simulink model "sampleModel1679"  (R2023a)
settings: Solver=VariableStepAuto  StartTime=0.0  StopTime=10.0  RelTol=1e-3
libraries: hdlsllib x5, simulink x2
settings Model: Creator=user1  LastModifiedBy=user1

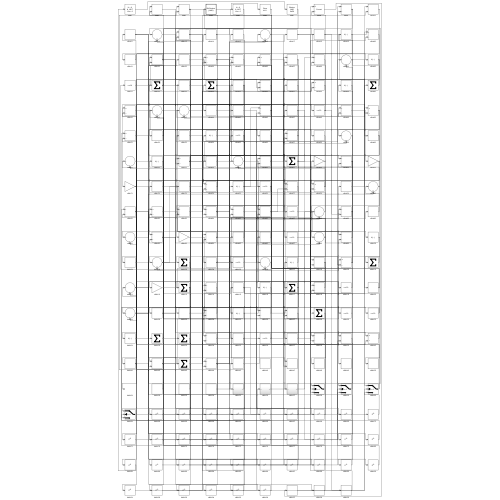
[thumbnail: Simulink's stored preview of the top-level diagram]
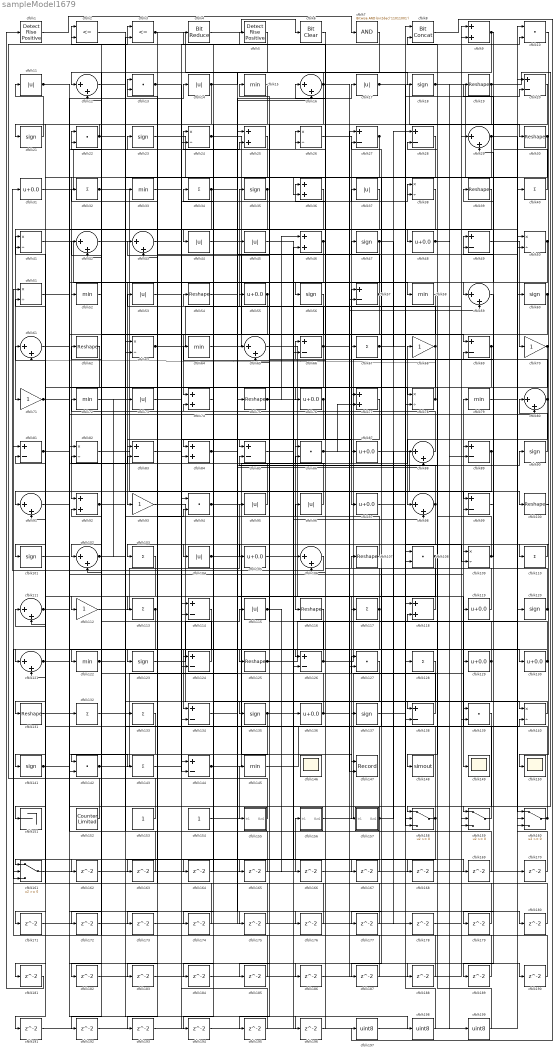
== system sampleModel1679 ==
  cfblk1 : hdlsllib/Logic and Bit Operations/Detect Rise Positive  vinit=0  OutDataTypeStr=boolean
  cfblk{10,13,22,86,94,108,127,139,142} (9 alike) : DotProduct  OutDataTypeStr=Inherit: Inherit via internal rule
  cfblk{19,30,39,54,62,75,100,107,116,125,131} (11 alike) : Reshape
  cfblk{18,21,23,35,47,56,60,90,101,120,123,135,137,141} (14 alike) : Signum
  cfblk{12,16,29,42..43,59,61,65,80,88,91,98,102,106,111,121} (16 alike) : Sum  Inputs=|++
  cfblk{32,34,40,67,103,110,113,117,128,132..133,143} (12 alike) : Sum  Inputs=+
  cfblk{11,14,17,37,44..45,53,73,95..96,104,115} (12 alike) : Abs  SaturateOnIntegerOverflow=off
  cfblk{31,48,55,76,87,97,105,119,129..130,136} (11 alike) : Bias  Bias=0.0  SaturateOnIntegerOverflow=off
  cfblk{24,26,38,41,50..51,63,78,82,109,140} (11 alike) : Product  Inputs=*/  RndMeth=Zero  SaturateOnIntegerOverflow=on
  cfblk{68,70..71,93,112} (5 alike) : Gain
  cfblk{20,27..28,49,57,66,69,81,83,85,89,99,114,124,126,134,138,144} (18 alike) : Sum  Inputs=+-
  cfblk{9,25,36,46,74,77,84,92,118} (9 alike) : Sum
  cfblk{15,33,52,58,64,72,79,122,145} (9 alike) : MinMax
  cfblk146 : Scope
      settings: Floating=on
  cfblk147 : Record  FileSettingsInternal="{\"entries\":[{\"content\":{\"excelSettings\":{\"content\":{},\"type\":\"Streamout.ExcelSettings\"}},\"type\":\"Streamout.FileSettingStorage\",\"uuid\":\"\"}],\"packageUris\":[\"http:\\/\\/schema.mathworks.com\\/mf0\\/streamout_blocks\\/R2020a\"],\"version\":\"1.0\"}"  Layout=[1 1]  SignalsInternal="{\"entries\":[{\"content\":{\"signals\":[{\"content\":{\"blockPath\":[],\"dimensions\":[1],\"domain\":\"\",\"lineColor\":\"#a2142f\",\"plots\":[1],\"port\":1,\"signalID\":2869,\"signalName\":\"XY Graph:1\"},\"type\":\"RecordBlkView.Signal\",\"uuid\":\"\"},{\"content\":{\"blockPath\":[],\"dimensions\":[1],\"domain\":\"\",\"lineColor\":\"#139fff\",\"plots\":[1],\"port\":2,\"signalID\":2872,\"signalName\":\"XY Graph:2\"},\"type\":\"RecordBlkView.Signal\",\"uuid\":\"\"}]},\"type\":\"RecordBlkView.InputSignals\",\"uuid\":\"\"}],\"packageUris\":[\"http:\\/\\/schema.mathworks.com\\/mf0\\/streamout_blocks\\/R2020a\"],\"version\":\"1.0\"}"  VisualizationBindings="{\"xyplotplugin\":{\"info\":[{\"series\":[{\"bindingParametersList\":[{\"parameter\":\"X-Axis\",\"signalID\":2869,\"signalName\":\"XY Graph:1\"},{\"parameter\":\"Y-Axis\",\"signalID\":2872,\"signalName\":\"XY Graph:2\"}],\"seriesID\":21956}],\"subplotID\":1}]}}"  CompatibilityTag=XY  st=-1
  cfblk148 : ToWorkspace  VariableName=simout  SaveFormat=Timeseries  SampleTime=-1
  cfblk149 : Scope
  cfblk150 : Scope
  cfblk151 : Terminator
  cfblk152 : hdlsllib/Sources/Counter Limited  uplimit=7  tsamp=-1
  cfblk153 : Constant  SampleTime=-1
  cfblk154 : Constant  SampleTime=-1
  cfblk155 : Subsystem
      settings: LibrarySourceBlock=|
      | hdlsllib/Ports &
      | Subsystems/Subsystem
  cfblk156 : Subsystem
      settings: LibrarySourceBlock=|
      | hdlsllib/Ports &
      | Subsystems/Subsystem
  cfblk157 : Subsystem
      settings: LibrarySourceBlock=|
      | hdlsllib/Ports &
      | Subsystems/Subsystem
  cfblk{158..161} (4 alike) : Switch  SaturateOnIntegerOverflow=off  InputSameDT=off
  cfblk{162..196} (35 alike) : Delay  SampleTime=1
  cfblk197 : DataTypeConversion  OutDataTypeStr=uint8  SaturateOnIntegerOverflow=off  RndMeth=Floor
  cfblk198 : DataTypeConversion  OutDataTypeStr=uint8  SaturateOnIntegerOverflow=off  RndMeth=Floor
  cfblk199 : DataTypeConversion  OutDataTypeStr=uint8  SaturateOnIntegerOverflow=off  RndMeth=Floor
  cfblk2 : RelationalOperator  Operator=<=  OutDataTypeStr=boolean  InputSameDT=off
  cfblk3 : RelationalOperator  Operator=<=  OutDataTypeStr=boolean  InputSameDT=off
  cfblk4 : hdlsllib/Logic and Bit Operations/Bit Reduce  mode=AND
  cfblk5 : hdlsllib/Logic and Bit Operations/Detect Rise Positive  vinit=0  OutDataTypeStr=boolean
  cfblk6 : simulink/Logic and Bit Operations/Bit Clear  iBit=0
      settings: LibrarySourceBlock=|
      | hdlsllib/Logic and Bit
      | Operations/Bit Clear
  cfblk7 : simulink/Logic and Bit Operations/Bitwise Operator  logicop=AND  UseBitMask=on  BitMask=bin2dec('11011001')  BitMaskRealWorld=Stored Integer
      settings: LibrarySourceBlock=|
      | hdlsllib/Logic and Bit
      | Operations/Bitwise
      | Operator
  cfblk8 : hdlsllib/Logic and Bit Operations/Bit Concat  numInputs=2
  wires:
  cfblk25/1 -> cfblk92/1
  cfblk30/1 -> cfblk43/2, cfblk171/1
  cfblk140/1 -> cfblk138/1
  cfblk24/1 -> cfblk69/1, cfblk119/1
  cfblk37/1 -> cfblk44/1
  cfblk46/1 -> cfblk93/1, cfblk26/1
  cfblk35/1 -> cfblk71/1, cfblk131/1, cfblk191/1
  cfblk36/1 -> cfblk102/1
  cfblk126/1 -> cfblk39/1, cfblk55/1
  cfblk100/1 -> cfblk150/1
  cfblk106/1 -> cfblk31/1
  cfblk76/1 -> cfblk85/1, cfblk193/1
  cfblk26/1 -> cfblk97/1
  cfblk107/1 -> cfblk13/1
  cfblk50/1 -> cfblk52/1, cfblk195/1
  cfblk156/1(Out1) -> cfblk79/1
  cfblk113/1 -> cfblk123/1, cfblk161/3
  cfblk155/1(Out1) -> cfblk3/1
  cfblk77/1 -> cfblk116/1
  cfblk20/1 -> cfblk84/1
  cfblk19/1 -> cfblk158/1, cfblk127/2
  cfblk118/1 -> cfblk2/1
  cfblk94/1 -> cfblk57/1, cfblk4/1
  cfblk114/1 -> cfblk134/1
  cfblk110/1 -> cfblk103/1
  cfblk74/1 -> cfblk34/1
  cfblk121/1 -> cfblk109/1, cfblk83/2, cfblk186/1
  cfblk66/1 -> cfblk35/1, cfblk124/2, cfblk49/2
  cfblk144/1 -> cfblk68/1, cfblk88/2, cfblk16/2
  cfblk81/1 -> cfblk158/3, cfblk175/1
  cfblk4/1 -> cfblk6/1
  cfblk109/1 -> cfblk85/2, cfblk49/1
  cfblk87/1 -> cfblk99/1
  cfblk75/1 -> cfblk149/1, cfblk46/1
  cfblk49/1 -> cfblk70/1
  cfblk90/1 -> cfblk80/1
  cfblk141/1 -> cfblk180/1, cfblk181/1
  cfblk5/1 -> cfblk102/2
  cfblk135/1 -> cfblk142/1, cfblk167/1
  cfblk43/1 -> cfblk58/1
  cfblk23/1 -> cfblk160/1
  cfblk72/1 -> cfblk144/1
  cfblk18/1 -> cfblk120/1, cfblk89/2
  cfblk102/1 -> cfblk3/2, cfblk73/1, cfblk126/2
  cfblk62/1 -> cfblk91/1
  cfblk1/1 -> cfblk7/1
  cfblk69/1 -> cfblk148/1, cfblk179/1
  cfblk65/1 -> cfblk157/1(In1)
  cfblk96/1 -> cfblk54/1
  cfblk161/1 -> cfblk156/1(In1)
  cfblk101/1 -> cfblk132/1
  cfblk145/1 -> cfblk99/2
  cfblk131/1 -> cfblk80/2
  cfblk31/1 -> cfblk23/1
  cfblk97/1 -> cfblk118/1
  cfblk139/1 -> cfblk159/1
  cfblk112/1 -> cfblk95/1
  cfblk60/1 -> cfblk113/1, cfblk138/2
  cfblk104/1 -> cfblk147/1, cfblk90/1
  cfblk142/1 -> cfblk45/1, cfblk169/1
  cfblk93/1 -> cfblk140/1
  cfblk32/1 -> cfblk144/2, cfblk12/2
  cfblk63/1 -> cfblk9/2, cfblk10/2
  cfblk134/1 -> cfblk75/1
  cfblk41/1 -> cfblk136/1
  cfblk125/1 -> cfblk40/1, cfblk185/1
  cfblk91/1 -> cfblk14/1
  cfblk17/1 -> cfblk30/1, cfblk109/2
  cfblk34/1 -> cfblk56/1, cfblk114/2
  cfblk29/1 -> cfblk60/1, cfblk147/2
  cfblk143/1 -> cfblk37/1
  cfblk6/1 -> cfblk86/1
  cfblk108/1 -> cfblk121/1, cfblk187/1
  cfblk115/1 -> cfblk165/1, cfblk166/1
  cfblk16/1 -> cfblk12/1, cfblk59/2, cfblk65/2
  cfblk89/1 -> cfblk69/2, cfblk158/2, cfblk141/1
  cfblk68/1 -> cfblk108/2, cfblk16/1
  cfblk127/1 -> cfblk137/1
  cfblk158/1 -> cfblk96/1, cfblk177/1
  cfblk80/1 -> cfblk98/1, cfblk43/1
  cfblk27/1 -> cfblk111/2, cfblk183/1
  cfblk44/1 -> cfblk17/1
  cfblk70/1 -> cfblk91/2, cfblk182/1
  cfblk57/1 -> cfblk74/1, cfblk32/1
  cfblk10/1 -> cfblk110/1
  cfblk92/1 -> cfblk133/1, cfblk94/2
  cfblk64/1 -> cfblk20/1
  cfblk130/1 -> cfblk125/1, cfblk66/1
  cfblk124/1 -> cfblk62/1
  cfblk123/1 -> cfblk115/1
  cfblk122/1 -> cfblk129/1, cfblk196/1
  cfblk11/1 -> cfblk126/1, cfblk67/1, cfblk48/1
  cfblk28/1 -> cfblk117/1
  cfblk138/1 -> cfblk42/1
  cfblk83/1 -> cfblk38/1
  cfblk15/1 -> cfblk101/1
  cfblk53/1 -> cfblk84/2
  cfblk119/1 -> cfblk5/1
  cfblk154/1 -> cfblk145/1
  cfblk73/1 -> cfblk76/1
  cfblk95/1 -> cfblk82/2
  cfblk132/1 -> cfblk140/2
  cfblk38/1 -> cfblk105/1
  cfblk79/1 -> cfblk10/1
  cfblk47/1 -> cfblk142/2, cfblk178/1
  cfblk152/1 -> cfblk61/1
  cfblk22/1 -> cfblk135/1, cfblk21/1, cfblk36/2
  cfblk55/1 -> cfblk83/1, cfblk184/1
  cfblk137/1 -> cfblk20/2
  cfblk117/1 -> cfblk86/2, cfblk121/2, cfblk24/1, cfblk194/1
  cfblk159/1 -> cfblk107/1
  cfblk40/1 -> cfblk19/1
  cfblk33/1 -> cfblk87/1
  cfblk78/1 -> cfblk61/2, cfblk36/1
  cfblk82/1 -> cfblk106/1
  cfblk39/1 -> cfblk104/1
  cfblk157/1(Out1) -> cfblk88/1, cfblk81/2, cfblk174/1
  cfblk3/1 -> cfblk65/1, cfblk173/1
  cfblk84/1 -> cfblk155/1(In1), cfblk47/1
  cfblk51/1 -> cfblk78/1
  cfblk14/1 -> cfblk151/1, cfblk18/1
  cfblk88/1 -> cfblk42/2
  cfblk67/1 -> cfblk130/1, cfblk28/1
  cfblk21/1 -> cfblk11/1
  cfblk129/1 -> cfblk139/1, cfblk15/1
  cfblk7/1 -> cfblk63/2
  cfblk99/1 -> cfblk29/2
  cfblk52/1 -> cfblk22/1
  cfblk42/1 -> cfblk128/1
  cfblk136/1 -> cfblk89/1, cfblk72/1
  cfblk9/1 -> cfblk112/1, cfblk59/1
  cfblk98/1 -> cfblk27/2, cfblk124/1
  cfblk105/1 -> cfblk98/2
  cfblk61/1 -> cfblk25/2
  cfblk103/1 -> cfblk122/1
  cfblk111/1 -> cfblk143/1, cfblk198/1
  cfblk71/1 -> cfblk41/1, cfblk190/1
  cfblk48/1 -> cfblk28/2, cfblk199/1
  cfblk153/1 -> cfblk41/2
  cfblk2/1 -> cfblk33/1
  cfblk160/1 -> cfblk51/2, cfblk127/1
  cfblk120/1 -> cfblk64/1, cfblk53/1
  cfblk85/1 -> cfblk100/1
  cfblk13/1 -> cfblk50/2, cfblk77/1
  cfblk86/1 -> cfblk38/2, cfblk77/2
  cfblk133/1 -> cfblk162/1
  cfblk162/1 -> cfblk160/2
  cfblk56/1 -> cfblk163/1
  cfblk163/1 -> cfblk63/1
  cfblk128/1 -> cfblk164/1
  cfblk164/1 -> cfblk74/2
  cfblk165/1 -> cfblk82/1
  cfblk166/1 -> cfblk78/2
  cfblk167/1 -> cfblk161/1
  cfblk45/1 -> cfblk168/1
  cfblk168/1 -> cfblk118/2
  cfblk169/1 -> cfblk92/2
  cfblk170/1 -> cfblk50/1
  cfblk171/1 -> cfblk25/1
  cfblk58/1 -> cfblk172/1
  cfblk172/1 -> cfblk29/1
  cfblk173/1 -> cfblk27/1
  cfblk174/1 -> cfblk51/1
  cfblk175/1 -> cfblk13/2
  cfblk54/1 -> cfblk176/1
  cfblk176/1 -> cfblk81/1
  cfblk177/1 -> cfblk114/1
  cfblk178/1 -> cfblk159/3
  cfblk179/1 -> cfblk9/1
  cfblk180/1 -> cfblk111/1
  cfblk181/1 -> cfblk1/1
  cfblk182/1 -> cfblk139/2
  cfblk183/1 -> cfblk46/2
  cfblk184/1 -> cfblk57/2
  cfblk185/1 -> cfblk22/2
  cfblk186/1 -> cfblk108/1
  cfblk187/1 -> cfblk161/2
  cfblk12/1 -> cfblk188/1
  cfblk188/1 -> cfblk2/2
  cfblk59/1 -> cfblk189/1
  cfblk189/1 -> cfblk159/2
  cfblk190/1 -> cfblk26/2
  cfblk191/1 -> cfblk66/2
  cfblk116/1 -> cfblk192/1
  cfblk192/1 -> cfblk134/2
  cfblk193/1 -> cfblk24/2
  cfblk194/1 -> cfblk160/3
  cfblk195/1 -> cfblk94/1
  cfblk196/1 -> cfblk106/2
  cfblk8/1 -> cfblk197/1
  cfblk197/1 -> cfblk170/1
  cfblk198/1 -> cfblk8/1
  cfblk199/1 -> cfblk8/2

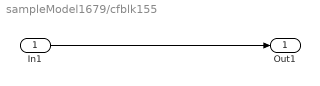
== system sampleModel1679/cfblk155 ==
  In1 : Inport
  Out1 : Outport
  wires:
  In1/1 -> Out1/1

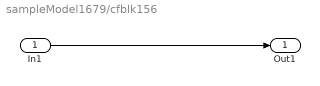
== system sampleModel1679/cfblk156 ==
  In1 : Inport
  Out1 : Outport
  wires:
  In1/1 -> Out1/1

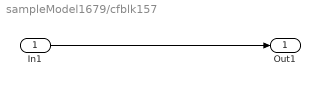
== system sampleModel1679/cfblk157 ==
  In1 : Inport
  Out1 : Outport
  wires:
  In1/1 -> Out1/1
